simulink library "SEMACE3_OUT"  (R2021b)
settings: Solver=VariableStepAuto  StartTime=0.0  StopTime=10.0  RelTol=1e-3
settings Model: Creator=ACH  LastModifiedBy=C83127

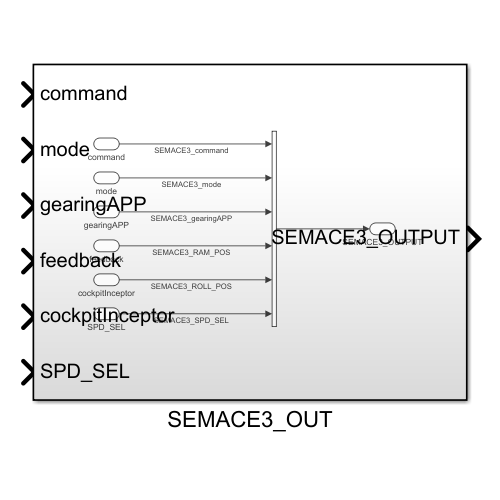
[thumbnail: Simulink's stored preview of the top-level diagram]
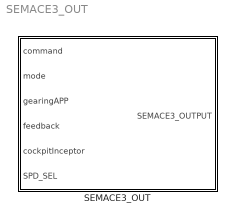
== system SEMACE3_OUT ==
  SEMACE3_OUT : Subsystem

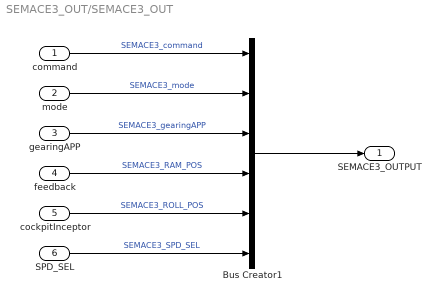
== system SEMACE3_OUT/SEMACE3_OUT ==
  command : Inport
  mode : Inport  Port=2
  gearingAPP : Inport  Port=3
  feedback : Inport  Port=4
  cockpitInceptor : Inport  Port=5
  SPD_SEL : Inport  Port=6
  Bus Creator1 : BusCreator  Inputs=6  OutDataTypeStr=Bus: SEMACE3_OUTPUT
  SEMACE3_OUTPUT : Outport  OutDataTypeStr=Bus: SEMACE3_OUTPUT
  wires:
  command/1 -> Bus Creator1/1  "SEMACE3_command"
  mode/1 -> Bus Creator1/2  "SEMACE3_mode"
  Bus Creator1/1 -> SEMACE3_OUTPUT/1
  gearingAPP/1 -> Bus Creator1/3  "SEMACE3_gearingAPP"
  feedback/1 -> Bus Creator1/4  "SEMACE3_RAM_POS"
  cockpitInceptor/1 -> Bus Creator1/5  "SEMACE3_ROLL_POS"
  SPD_SEL/1 -> Bus Creator1/6  "SEMACE3_SPD_SEL"
